simulink model "task5"  (R2020a)
settings: Solver=VariableStepAuto  StartTime=0.0  StopTime=10  RelTol=1e-3
undefined symbols (not defined in the file or in its folder): nofriction, p560, transl, troty
libraries: roblocks x9
settings Model: Creator=root  LastModifiedBy=root

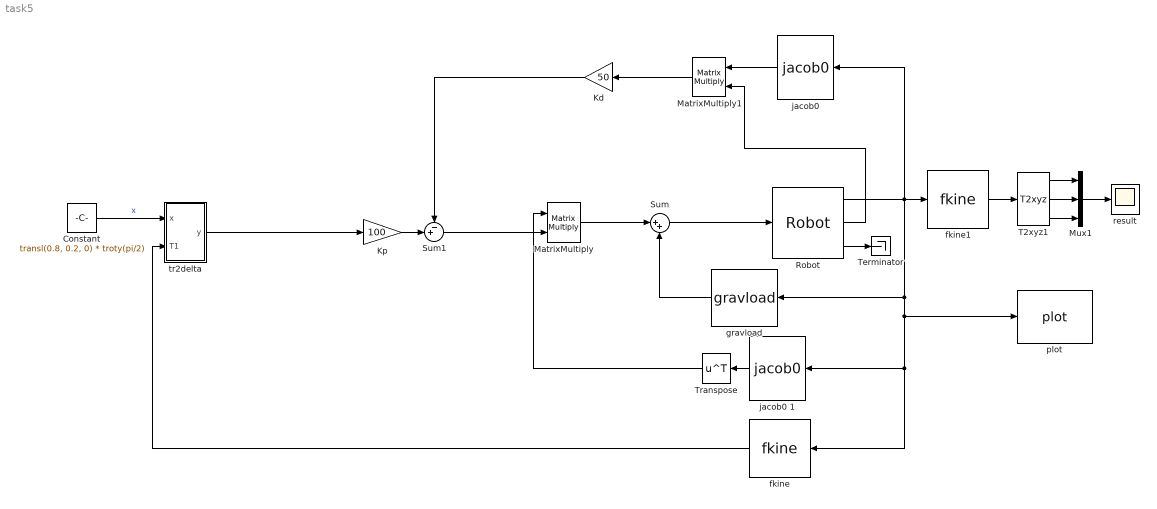
== system task5 ==
  Constant : Constant  Value=transl(0.8, 0.2, 0) * troty(pi/2)
  Kd : Gain  Gain=50
  Kp : Gain  Gain=100
  MatrixMultiply : Product  Multiplication=Matrix(*)
  MatrixMultiply1 : Product  Multiplication=Matrix(*)
  Mux1 : Mux  Inputs=3
  Robot : roblocks/Arm/Robot  robot=nofriction(p560)  q0=[0 0 0 0 0 0]
  Sum : Sum  Inputs=|++
  Sum1 : Sum  Inputs=-+|
  T2xyz1 : roblocks/Toolbox/T2xyz
  Terminator : Terminator
  Transpose : Math  Operator=transpose  SaturateOnIntegerOverflow=on
  fkine : roblocks/Arm/fkine  robot=nofriction(p560)
  fkine1 : roblocks/Arm/fkine  robot=nofriction(p560)
  gravload : roblocks/Arm/gravload  robot=nofriction(p560)
  "jacob0 " : roblocks/Arm/jacob0   robot=nofriction(p560)
  jacob0 1 : roblocks/Arm/jacob0   robot=nofriction(p560)
  plot : roblocks/Arm/plot  robot=nofriction(p560)  fps=5  holdplot=on
  result : Scope
  tr2delta : Subsystem
  wires:
  Robot/1 -> fkine1/1, "jacob0 "/1, gravload/1, plot/1, fkine/1, jacob0 1/1
  Kp/1 -> Sum1/2
  "jacob0 "/1 -> MatrixMultiply1/1
  Kd/1 -> Sum1/1
  jacob0 1/1 -> Transpose/1
  MatrixMultiply/1 -> Sum/1
  Transpose/1 -> MatrixMultiply/1
  gravload/1 -> Sum/2
  Sum/1 -> Robot/1
  T2xyz1/1 -> Mux1/1
  T2xyz1/2 -> Mux1/2
  T2xyz1/3 -> Mux1/3
  fkine1/1 -> T2xyz1/1
  Mux1/1 -> result/1
  Robot/3 -> Terminator/1
  MatrixMultiply1/1 -> Kd/1
  Robot/2 -> MatrixMultiply1/2
  Sum1/1 -> MatrixMultiply/2
  Constant/1 -> tr2delta/1(x)  "x"
  fkine/1 -> tr2delta/2(T1)
  tr2delta/1(y) -> Kp/1

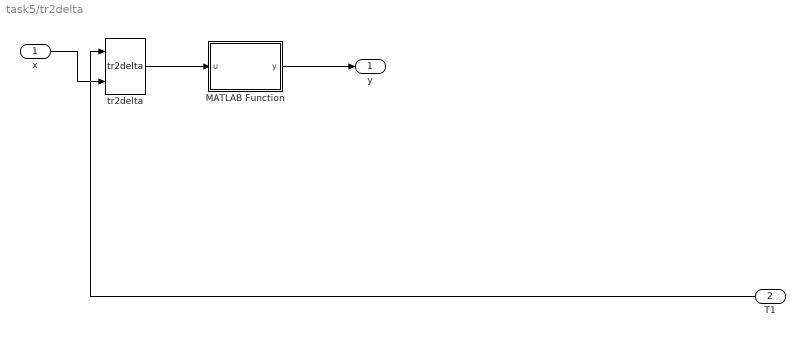
== system task5/tr2delta ==
  x : Inport
  T1 : Inport  Port=2
  MATLAB Function : MATLAB Function  TreatAsAtomicUnit=on
  tr2delta : roblocks/Toolbox/tr2delta
  y : Outport
  wires:
  tr2delta/1 -> MATLAB Function/1(u)
  MATLAB Function/1(y) -> y/1
  T1/1 -> tr2delta/1
  x/1 -> tr2delta/2

== matlab function task5/tr2delta/MATLAB Function ==
  data: u input; y output
function y = fcn(u)

t = u(1);
u(1) = u(3);
u(3) = -1*t;

y = u;
